simulink model "Pcontroller"  (R2021b)
settings: Solver=VariableStepAuto  StartTime=0.0  StopTime=20  RelTol=1e-3
model workspace (MAT data in the model file):
  L = 0.2
values from neighbouring files (symbols this model uses):
  Td = 100e-6    (= 0.0001)    [simConstants.m]
  theta0 = deg2rad(5)    [simConstants.m]
libraries: simulink_extras x1
settings Model: PacingRate=1.100000  Creator=logan  LastModifiedBy=logan

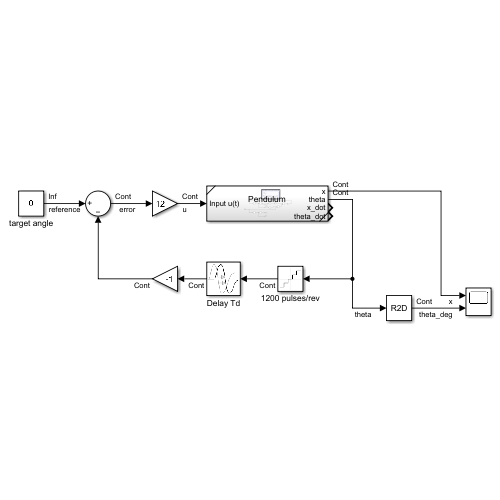
[thumbnail: Simulink's stored preview of the top-level diagram]
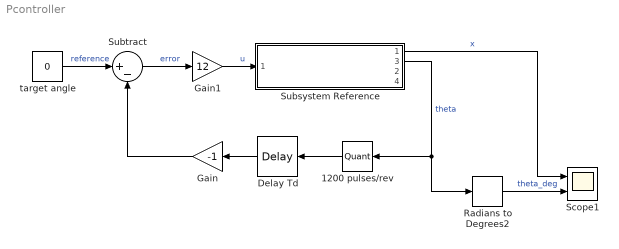
== system Pcontroller ==
  1200 pulses/rev : Quantizer  QuantizationInterval=(2*pi)/1200
  Delay Td : TransportDelay  DelayTime=Td  InitialOutput=theta0
  Gain : Gain  Gain=-1
  Gain1 : Gain  Gain=12
  Radians to Degrees2 : simulink_extras/Transformations/Radians to Degrees
  Scope1 : Scope  NumInputPorts=2
  Subsystem Reference : Subsystem  ReferencedSubsystem=Pendulum
      settings: PortSchema="{\"entries\":[{\"content\":{\"sides\":[{\"content\":{\"connectorIds\":[\"In1\"]},\"type\":\"ConnectorPlacement.EquallySpacedRectSide\",\"uuid\":\"caec1104-e2e6-4c31-8105-8fc922dae5e8\"},{\"content\":{\"connectorIds\":[\"Out1\",\"Out3\",\"Out2\",\"Out4\"],\"side\":\"RIGHT\"},\"type\":\"ConnectorPlacement.EquallySpacedRectSide\",\"uuid\":\"5fd37d83-c645-402c-ac25-1888ccf1b1a6\"},{\"content\":{\"connectorIds\":[],\"side\":\"TOP\"},\"type\":\"ConnectorPlacement.EquallySpacedRectSide\",\"uuid\":\"2e43f1c0-40e6-4dcf-a44e-f71c6f7202b4\"}]},\"type\":\"ConnectorPlacement.EquallySpacedConnector\",\"uuid\":\"6200bc17-7860-41df-9508-8c7d9814e84e\"}],\"packageUris\":[\"http://schema.mathworks.com/mf0/Connector/R2020b\"],\"version\":\"1.0\"}"
  Subtract : Sum  Inputs=|+-
  target angle : Constant  Value=0  OutDataTypeStr=Inherit: Inherit via back propagation
  wires:
  Subsystem Reference/1 -> Scope1/1  "x"
  Gain1/1 -> Subsystem Reference/1  "u"
  Subsystem Reference/3 -> 1200 pulses/rev/1, Radians to Degrees2/1  "theta"
  Subtract/1 -> Gain1/1  "error"
  Gain/1 -> Subtract/2
  target angle/1 -> Subtract/1  "reference"
  Radians to Degrees2/1 -> Scope1/2  "theta_deg"
  1200 pulses/rev/1 -> Delay Td/1
  Delay Td/1 -> Gain/1
